simulink model "untitled"  (R2023b)
settings: Solver=VariableStepAuto  StartTime=0.0  StopTime=10.0  RelTol=1e-3
settings Model: Creator=alberto  LastModifiedBy=alberto

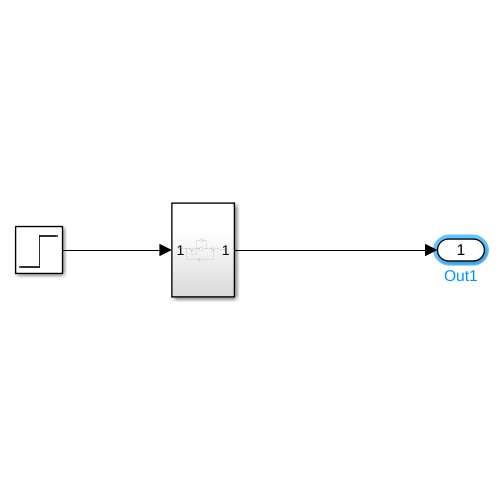
[thumbnail: Simulink's stored preview of the top-level diagram]
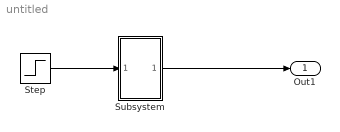
== system untitled ==
  Step : Step  SampleTime=0
  Subsystem : Subsystem
  Out1 : Outport
  wires:
  Subsystem/1(Out1) -> Out1/1
  Step/1 -> Subsystem/1(In1)

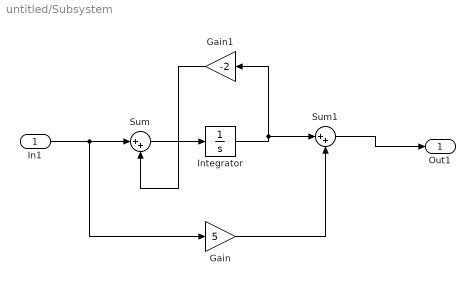
== system untitled/Subsystem ==
  In1 : Inport
  Gain : Gain  Gain=5
  Gain1 : Gain  Gain=-2
  Integrator : Integrator
  Sum : Sum  Inputs=|++
  Sum1 : Sum  Inputs=|++
  Out1 : Outport
  wires:
  Sum/1 -> Integrator/1
  Gain/1 -> Sum1/2
  Gain1/1 -> Sum/2
  Sum1/1 -> Out1/1
  Integrator/1 -> Sum1/1, Gain1/1
  In1/1 -> Gain/1, Sum/1
